simulink model "simple_ex01"  (Simulink 7.6)
settings: Solver=ode45  StartTime=0.0  StopTime=10.0  RelTol=1e-3
PreLoadFcn:
  | ParamA = 2;
  | ParamB = 3;
undefined symbols (not defined in the file): sldvsubsys
libraries: sldvlib x13, simulink x1, propertySpecificationOperatorLib x1
settings Model: Creator=itoy  LastModifiedBy=itoy

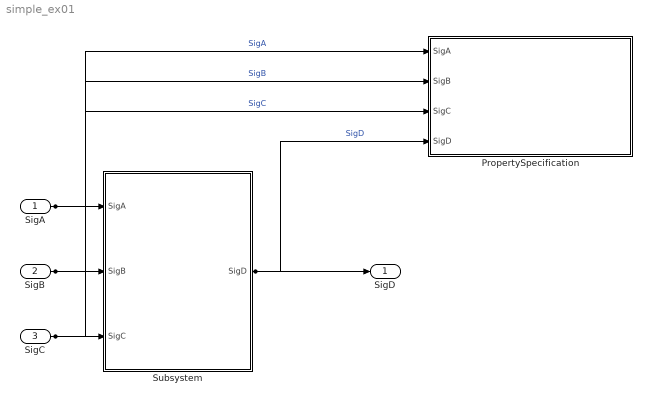
== system simple_ex01 ==
  SigA : Inport
  SigB : Inport  Port=2
  SigC : Inport  Port=3
  PropertySpecification : Subsystem  Tag=VerificationSubsystem  DisableCoverage=on  LoadFcn=sldvsubsys('check')  TreatAsAtomicUnit=on  SimViewingDevice=on  mask(VerificationSubsystem){}
      mask help: Property Specification Block
      mask init:
      | sldvsubsys('maskInit');
      settings: OpenFcn=PropertySpecificationUI('Block',gcb)
      settings: CopyFcn=|
      | sldvsubsys('copy');
      |  set_param(gcb,'LinkStatus','none')
      settings: PreSaveFcn=|
      | set_param(gcb,'SimViewingDevice','on');
      | sldvsubsys('check');
      mask Help: helpview(fullfile(docroot,'toolbox','sldv','sldv.map'),'verificationsubsystem')
      mask Display: image(imread('sldvicon_versubsys.png','BackGroundColor',[1 1 1]),'center');
  Subsystem : Subsystem
  SigD : Outport
  wires:
  SigA/1 -> Subsystem/1(SigA), PropertySpecification/1(SigA)  "SigA"
  SigB/1 -> Subsystem/2(SigB), PropertySpecification/2(SigB)  "SigB"
  SigC/1 -> Subsystem/3(SigC), PropertySpecification/3(SigC)  "SigC"
  Subsystem/1(SigD) -> SigD/1, PropertySpecification/4(SigD)  "SigD"

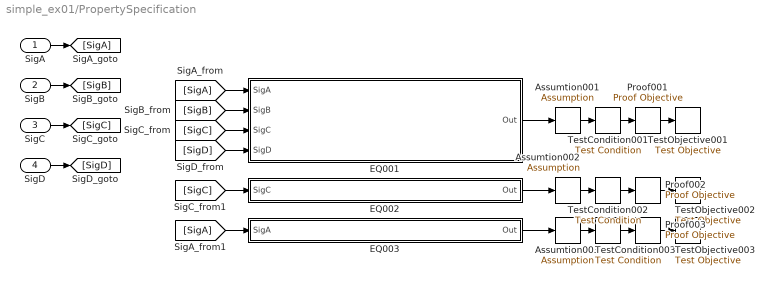
== system simple_ex01/PropertySpecification ==
  SigA : Inport
  SigB : Inport  Port=2
  SigC : Inport  Port=3
  SigD : Inport  Port=4
  Assumtion001 : sldvlib/Assumption  SystemSampleTime=-1  enabled=off  customAVTBlockType=Assumption  intervals=true  initial=off  dispValues=on  outEnabled=on
      settings: AttributesFormatString=%<intervals>
  Assumtion002 : sldvlib/Assumption  SystemSampleTime=-1  enabled=off  customAVTBlockType=Assumption  intervals=true  initial=off  dispValues=on  outEnabled=on
      settings: AttributesFormatString=%<intervals>
  Assumtion003 : sldvlib/Assumption  SystemSampleTime=-1  enabled=on  customAVTBlockType=Assumption  intervals=true  initial=off  dispValues=on  outEnabled=on
      settings: AttributesFormatString=%<intervals>
  EQ001 : Subsystem  Tag=CustomScope  mask(Equation2Simulink block){InputVar=SigA,SigB,SigC,SigD, ParamVar=ParamA,ParamB, VerifEq=SigA > 0 && ( SigB + SigC < ParamA) ==> SigD == ParamB}
      mask prompts: InputVar "入力変数"; ParamVar "パラメータ変数"; VerifEq "検査式"
      mask help: Equation2Simulink block
      mask init:
      | Equation2Simulink(VerifEq,gcb,InputVar,ParamVar);
      mask Display: disp(VerifEq)
  EQ002 : Subsystem  Tag=CustomScope  mask(Equation2Simulink block){InputVar=SigC, ParamVar=, VerifEq=SigC - prev(SigC,1) < 100}
      mask prompts: InputVar "入力変数"; ParamVar "パラメータ変数"; VerifEq "検査式"
      mask help: Equation2Simulink block
      mask init:
      | Equation2Simulink(VerifEq,gcb,InputVar,ParamVar);
      mask Display: disp(VerifEq)
  EQ003 : Subsystem  Tag=CustomScope  mask(Equation2Simulink block){InputVar=SigA, ParamVar=, VerifEq=init(SigA==3,2)}
      mask prompts: InputVar "入力変数"; ParamVar "パラメータ変数"; VerifEq "検査式"
      mask help: Equation2Simulink block
      mask init:
      | Equation2Simulink(VerifEq,gcb,InputVar,ParamVar);
      mask Display: disp(VerifEq)
  Proof001 : sldvlib/Proof Objective  SystemSampleTime=-1  enabled=on  customAVTBlockType=Proof Objective  intervals=true  dispValues=on  outEnabled=on  enableStopSim=off
      settings: AttributesFormatString=%<intervals>
  Proof002 : sldvlib/Proof Objective  SystemSampleTime=-1  enabled=on  customAVTBlockType=Proof Objective  intervals=true  dispValues=on  outEnabled=on  enableStopSim=off
      settings: AttributesFormatString=%<intervals>
  Proof003 : sldvlib/Proof Objective  SystemSampleTime=-1  enabled=off  customAVTBlockType=Proof Objective  intervals=true  dispValues=on  outEnabled=on  enableStopSim=off
      settings: AttributesFormatString=%<intervals>
  TestCondition001 : sldvlib/Test Condition  SystemSampleTime=-1  enabled=off  customAVTBlockType=Test Condition  intervals=true  initial=off  dispValues=on  outEnabled=on
      settings: AttributesFormatString=%<intervals>
  TestCondition002 : sldvlib/Test Condition  SystemSampleTime=-1  enabled=off  customAVTBlockType=Test Condition  intervals=true  initial=off  dispValues=on  outEnabled=on
      settings: AttributesFormatString=%<intervals>
  TestCondition003 : sldvlib/Test Condition  SystemSampleTime=-1  enabled=on  customAVTBlockType=Test Condition  intervals=true  initial=off  dispValues=on  outEnabled=on
      settings: AttributesFormatString=%<intervals>
  TestObjective001 : sldvlib/Test Objective  SystemSampleTime=-1  enabled=on  customAVTBlockType=Test Objective  intervals=true  dispValues=on  outEnabled=off
      settings: AttributesFormatString=%<intervals>
  TestObjective002 : sldvlib/Test Objective  SystemSampleTime=-1  enabled=on  customAVTBlockType=Test Objective  intervals=true  dispValues=on  outEnabled=off
      settings: AttributesFormatString=%<intervals>
  TestObjective003 : sldvlib/Test Objective  SystemSampleTime=-1  enabled=off  customAVTBlockType=Test Objective  intervals=true  dispValues=on  outEnabled=off
      settings: AttributesFormatString=%<intervals>
  wires:
  EQ001/1(Out) -> Assumtion001/1
  Assumtion001/1 -> TestCondition001/1
  TestCondition001/1 -> Proof001/1
  Proof001/1 -> TestObjective001/1
  [SigA] -> EQ001/1(SigA)
  [SigB] -> EQ001/2(SigB)
  [SigC] -> EQ001/3(SigC)
  [SigD] -> EQ001/4(SigD)
  EQ002/1(Out) -> Assumtion002/1
  Assumtion002/1 -> TestCondition002/1
  TestCondition002/1 -> Proof002/1
  Proof002/1 -> TestObjective002/1
  [SigC] -> EQ002/1(SigC)
  EQ003/1(Out) -> Assumtion003/1
  Assumtion003/1 -> TestCondition003/1
  TestCondition003/1 -> Proof003/1
  Proof003/1 -> TestObjective003/1
  [SigA] -> EQ003/1(SigA)
  SigA/1 -> [SigA]
  SigB/1 -> [SigB]
  SigC/1 -> [SigC]
  SigD/1 -> [SigD]

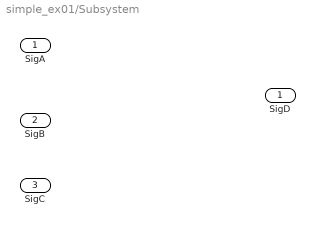
== system simple_ex01/Subsystem ==
  SigA : Inport
  SigB : Inport  Port=2
  SigC : Inport  Port=3
  SigD : Outport

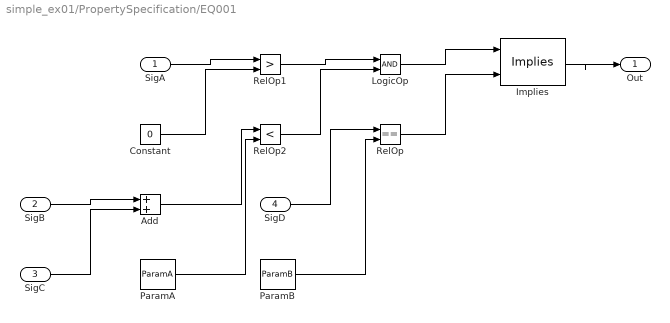
== system simple_ex01/PropertySpecification/EQ001 ==
  SigA : Inport
  SigB : Inport  Port=2
  SigC : Inport  Port=3
  SigD : Inport  Port=4
  Add : Sum  SaturateOnIntegerOverflow=on  InputSameDT=on  OutDataTypeStr=Inherit: Same as first input
  Constant : Constant  Value=0  OutDataTypeStr=Inherit: Inherit via back propagation
  Implies : sldvlib/Implies  SystemSampleTime=-1
  LogicOp : Logic
  ParamA : Constant  Value=ParamA
  ParamB : Constant  Value=ParamB
  RelOp : RelationalOperator  Operator===  InputSameDT=on
  RelOp1 : RelationalOperator  Operator=>  InputSameDT=on
  RelOp2 : RelationalOperator  Operator=<  InputSameDT=on
  Out : Outport
  wires:
  Implies/1 -> Out/1
  SigB/1 -> Add/1
  SigA/1 -> RelOp1/1
  RelOp1/1 -> LogicOp/1
  LogicOp/1 -> Implies/1
  SigC/1 -> Add/2
  RelOp/1 -> Implies/2
  SigD/1 -> RelOp/1
  RelOp2/1 -> LogicOp/2
  Constant/1 -> RelOp1/2
  Add/1 -> RelOp2/1
  ParamB/1 -> RelOp/2
  ParamA/1 -> RelOp2/2

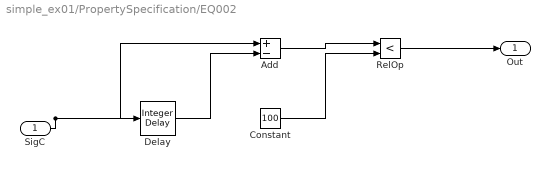
== system simple_ex01/PropertySpecification/EQ002 ==
  SigC : Inport
  Add : Sum  Inputs=+-  SaturateOnIntegerOverflow=on  InputSameDT=on  OutDataTypeStr=Inherit: Same as first input
  Constant : Constant  Value=100  OutDataTypeStr=Inherit: Inherit via back propagation
  Delay : simulink/Discrete/Integer Delay  NumDelays=1  vinit=0.0  samptime=-1
  RelOp : RelationalOperator  Operator=<  InputSameDT=on
  Out : Outport
  wires:
  SigC/1 -> Delay/1, Add/1
  RelOp/1 -> Out/1
  Add/1 -> RelOp/1
  Delay/1 -> Add/2
  Constant/1 -> RelOp/2

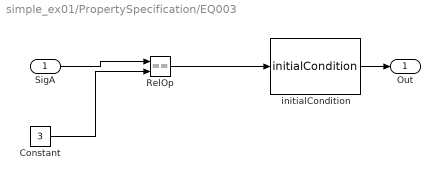
== system simple_ex01/PropertySpecification/EQ003 ==
  SigA : Inport
  Constant : Constant  Value=3  OutDataTypeStr=Inherit: Inherit via back propagation
  RelOp : RelationalOperator  Operator===  InputSameDT=on
  initialCondition : propertySpecificationOperatorLib/initialCondition  SystemSampleTime=-1  DelayCount=2
  Out : Outport
  wires:
  initialCondition/1 -> Out/1
  SigA/1 -> RelOp/1
  RelOp/1 -> initialCondition/1
  Constant/1 -> RelOp/2
